simulink model "testGrindingMachine"  (R2025a)
settings: Solver=VariableStepAuto  StartTime=0.0  StopTime=10.0  RelTol=1e-3
libraries: StdLib x11, ProductionLinePLib x1
settings Model: Creator=peter  LastModifiedBy=peter
settings RTWCC: GPUComputeCapability=3.5

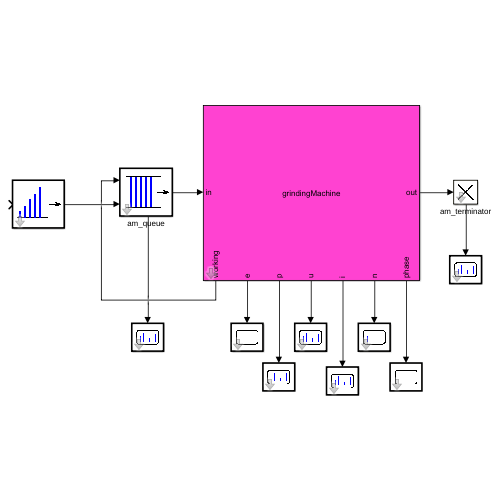
[thumbnail: Simulink's stored preview of the top-level diagram]
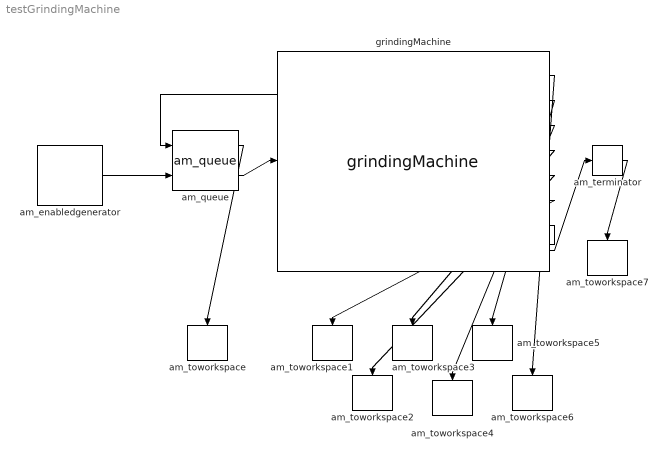
== system testGrindingMachine ==
  am_enabledgenerator : StdLib/am_enabledgenerator  tG=3000  n0=0  nG=4  tD=[0,2]  tau=[0,1]  debug=0
  am_queue : StdLib/am_queue  tD=[0,5]  tau=[0,5]  debug=0
  am_terminator : StdLib/am_terminator  tau=[0,1]  debug=0
  am_toworkspace : StdLib/am_toworkspace  varname="\"nq\""  t0=0  format="\"vector\""  tau=[0,5]  debug=0
  am_toworkspace1 : StdLib/am_toworkspace  varname="\"E\""  t0=0  format="\"vector\""  tau=[0,5]  debug=0
  am_toworkspace2 : StdLib/am_toworkspace  varname="\"P\""  t0=0  format="\"vector\""  tau=[0,5]  debug=0
  am_toworkspace3 : StdLib/am_toworkspace  varname="\"u\""  t0=0  format="\"vector\""  tau=[0,5]  debug=0
  am_toworkspace4 : StdLib/am_toworkspace  varname="\"i\""  t0=0  format="\"vector\""  tau=[0,5]  debug=0
  am_toworkspace5 : StdLib/am_toworkspace  varname="\"n\""  t0=0  format="\"vector\""  tau=[0,5]  debug=0
  am_toworkspace6 : StdLib/am_toworkspace  varname="\"phase\""  t0=0  format="\"vector\""  tau=[0,5]  debug=0
  am_toworkspace7 : StdLib/am_toworkspace  varname="\"nout\""  t0=0  format="\"vector\""  tau=[0,5]  debug=0
  grindingMachine : ProductionLinePLib/grindingMachine  grinding_time=27*60  vfr1_ug=0.48  vfr2_ug=0.19  vfr3_ug=0.03  vc_ug=30  vfr1_og=1.86  vfr2_og=0.53  vfr3_og=0.16  vc_og=50  P_vfr1=0.2  P_vfr2=0.2  P_vfr3=0.2  P_vc=0.6  vfr1=0.48  vfr2=0.19  vfr3=0.03  vc=30  tauInt=[0,100]  tauCont=[0,100]  tau=[0,1]  debug=0
      settings: LibrarySourceBlock=ProductionLineLib_CM/grinding
  wires:
  am_enabledgenerator/1 -> am_queue/1
  grindingMachine/1 -> am_terminator/1
  grindingMachine/2 -> am_queue/2
  am_queue/1 -> grindingMachine/1
  am_queue/2 -> am_toworkspace/1
  am_terminator/1 -> am_toworkspace7/1
  grindingMachine/3 -> am_toworkspace1/1
  grindingMachine/4 -> am_toworkspace2/1
  grindingMachine/5 -> am_toworkspace3/1
  grindingMachine/6 -> am_toworkspace4/1
  grindingMachine/7 -> am_toworkspace5/1
  grindingMachine/8 -> am_toworkspace6/1
